simulink subsystem "PieroHFz"  (R2023b)
settings: Solver=VariableStepAuto  StartTime=0.0  StopTime=10.0  RelTol=1e-3
settings Model: Creator=Hajar  LastModifiedBy=Hajar

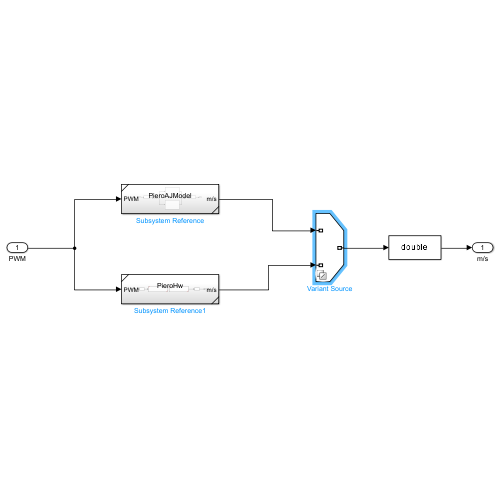
[thumbnail: Simulink's stored preview of the top-level diagram]
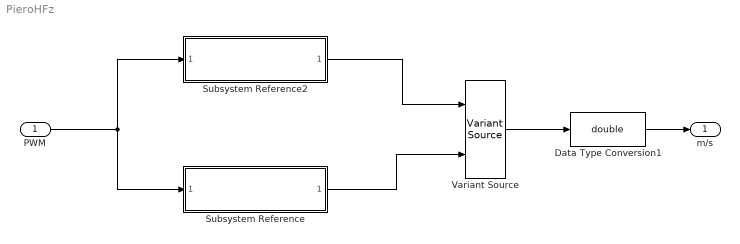
== system PieroHFz ==
  PWM : Inport
  Data Type Conversion1 : DataTypeConversion  OutDataTypeStr=double  SaturateOnIntegerOverflow=off  RndMeth=Floor
  Subsystem Reference : Subsystem  ReferencedSubsystem=PieroHwz
  Subsystem Reference2 : Subsystem  ReferencedSubsystem=PieroHFModelz
  Variant Source : VariantSource  VariantControlMode=sim codegen switching
  m/s : Outport
  wires:
  Data Type Conversion1/1 -> m/s/1
  PWM/1 -> Subsystem Reference2/1, Subsystem Reference/1
  Subsystem Reference2/1 -> Variant Source/1
  Subsystem Reference/1 -> Variant Source/2
  Variant Source/1 -> Data Type Conversion1/1
